simulink model "es_2_1"  (R2014a)
settings: Solver=ode45  StartTime=0.0  StopTime=120.0  RelTol=1e-3
values from neighbouring files (symbols this model uses):
  Kc = -0.1    [es2.m]
  Kr = 0.5    [es2.m]
libraries: cstblocks x1, simulink x1
settings Model: Creator=HP  LastModifiedBy=HP

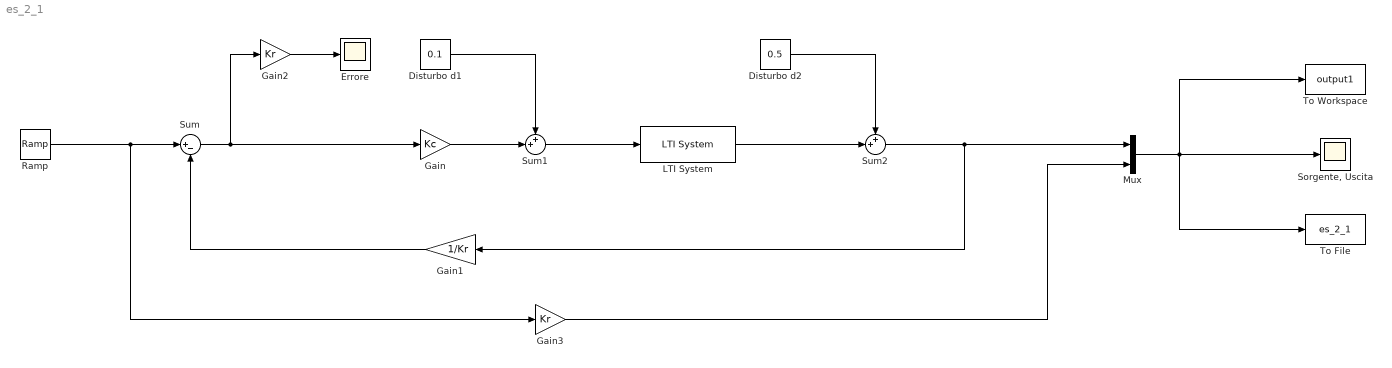
== system es_2_1 ==
  Disturbo d1 : Constant  Value=0.1
  Disturbo d2 : Constant  Value=0.5
  Errore : Scope
  Gain : Gain  Gain=Kc
  Gain1 : Gain  Gain=1/Kr
  Gain2 : Gain  Gain=Kr
  Gain3 : Gain  Gain=Kr
  LTI System : cstblocks/LTI System  sys=F  IC=[]
  Mux : Mux  Inputs=2
  Ramp : simulink/Sources/Ramp  slope=1  start=0  X0=0
  "Sorgente, Uscita" : Scope
  Sum : Sum  Inputs=|+-
  Sum1 : Sum  Inputs=++|
  Sum2 : Sum  Inputs=++|
  To File : ToFile  Filename=es_2_1  SaveFormat=Timeseries
  To Workspace : ToWorkspace  VariableName=output1  SaveFormat=Timeseries  SampleTime=-1
  wires:
  Ramp/1 -> Gain3/1, Sum/1
  Gain1/1 -> Sum/2
  Sum/1 -> Gain2/1, Gain/1
  Gain2/1 -> Errore/1
  Disturbo d1/1 -> Sum1/1
  Gain/1 -> Sum1/2
  Sum1/1 -> LTI System/1
  Disturbo d2/1 -> Sum2/1
  LTI System/1 -> Sum2/2
  Mux/1 -> To Workspace/1, To File/1, "Sorgente, Uscita"/1
  Sum2/1 -> Gain1/1, Mux/1
  Gain3/1 -> Mux/2
